simulink model "untitled"  (R2014b)
settings: Solver=ode45  StartTime=0.0  StopTime=10.0  RelTol=1e-3
settings Model: Creator=rajab  LastModifiedBy=rajab

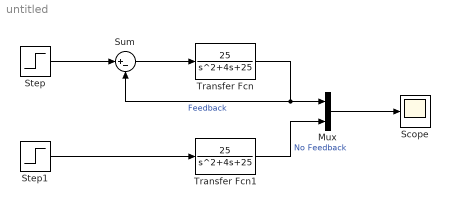
== system untitled ==
  Mux : Mux  Inputs=2
  Scope : Scope
      settings: ShowLegends=on
  Step : Step  SampleTime=0
  Step1 : Step  SampleTime=0
  Sum : Sum  Inputs=|+-
  Transfer Fcn : TransferFcn  Numerator=[25]  Denominator=[1 4 25]
  Transfer Fcn1 : TransferFcn  Numerator=[25]  Denominator=[1 4 25]
  wires:
  Step/1 -> Sum/1
  Sum/1 -> Transfer Fcn/1
  Transfer Fcn/1 -> Sum/2, Mux/1  "Feedback"
  Transfer Fcn1/1 -> Mux/2  "No Feedback"
  Step1/1 -> Transfer Fcn1/1
  Mux/1 -> Scope/1
